simulink model "MPC"  (R2020a)
settings: Solver=ode4  StartTime=0.0  StopTime=200  FixedStep=1  RelTol=1e-3
InitFcn:
  | SetupParameters
StopFcn:
  | PlotResults
values from neighbouring files (symbols this model uses):
  A = reshape(Aflat,n,n)    [mpc_s_L2.m]    (also in prediction.m = delayMod.A)
  B1 = reshape(B1flat,n,[])    [mpc_s_L2.m]    (also in prediction.m = delayMod.B1)
  CforStateOutput = eye(4)    [SetupParameters.m]    (also in TestMPC.m)
  DforStateOutput = zeros(n, p)    [SetupParameters.m]    (also in TestMPC.m)
  G = [G11 G12; G21 G22]    [SetupParameters.m]    (also in TestMPC.m)
  plantD = ss(Gd)    [SetupParameters.m]    (also in TestMPC.m; mpc_s_L2.m)
  tau = block.Dwork(11).Data    [mpc_s_L2.m]    (also in prediction.m = delayMod.tau)
  Ts = 1    [SetupParameters.m]    (also in TestMPC.m; mpc_s_L2.m = block.DialogPrm(8).Data)
undefined symbols (not defined in the file or in its folder): H
settings Model: Creator=Charl  LastModifiedBy=Charl

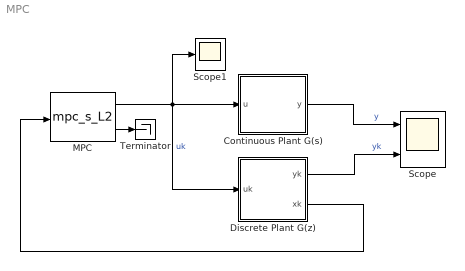
== system MPC ==
  Continuous Plant G(s) : Subsystem
  Discrete Plant G(z) : Subsystem
  MPC : M-S-Function  FunctionName=mpc_s_L2  Parameters=Gd, Ysp, Np, Nb, Nc, Q, R, Ts
  Scope : Scope  NumInputPorts=2
  Scope1 : Scope
  Terminator : Terminator
  wires:
  Continuous Plant G(s)/1(y) -> Scope/1  "y"
  MPC/1 -> Scope1/1, Discrete Plant G(z)/1(uk), Continuous Plant G(s)/1(u)  "uk"
  MPC/2 -> Terminator/1
  Discrete Plant G(z)/2(xk) -> MPC/1
  Discrete Plant G(z)/1(yk) -> Scope/2  "yk"

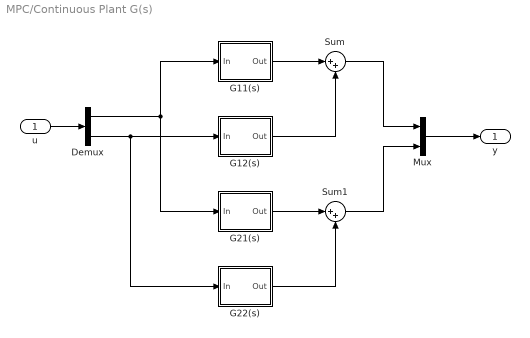
== system MPC/Continuous Plant G(s) ==
  u : Inport
  Demux : Demux  Outputs=2
  G11(s) : Subsystem
  G12(s) : Subsystem
  G21(s) : Subsystem
  G22(s) : Subsystem
  Mux : Mux  Inputs=2
  Sum : Sum  Inputs=|++
  Sum1 : Sum  Inputs=|++
  y : Outport
  wires:
  G11(s)/1(Out) -> Sum/1
  G22(s)/1(Out) -> Sum1/2
  G21(s)/1(Out) -> Sum1/1
  G12(s)/1(Out) -> Sum/2
  Demux/1 -> G11(s)/1(In), G21(s)/1(In)
  Demux/2 -> G22(s)/1(In), G12(s)/1(In)
  u/1 -> Demux/1
  Sum/1 -> Mux/1
  Sum1/1 -> Mux/2
  Mux/1 -> y/1

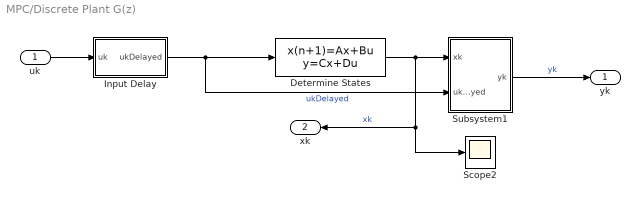
== system MPC/Discrete Plant G(z) ==
  uk : Inport
  Determine States : DiscreteStateSpace  A=A  B=B1  C=CforStateOutput  D=DforStateOutput  SampleTime=Ts
  Input Delay : Subsystem
  Scope2 : Scope
  Subsystem1 : Subsystem
  yk : Outport
  xk : Outport  Port=2
  wires:
  Input Delay/1(ukDelayed) -> Determine States/1, Subsystem1/2(ukDelayed)  "ukDelayed"
  uk/1 -> Input Delay/1(uk)
  Determine States/1 -> xk/1, Scope2/1, Subsystem1/1(xk)  "xk"
  Subsystem1/1(yk) -> yk/1  "yk"

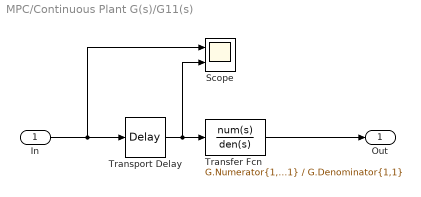
== system MPC/Continuous Plant G(s)/G11(s) ==
  In : Inport
  Scope : Scope  NumInputPorts=2
  Transfer Fcn : TransferFcn  Numerator=G.Numerator{1,1}  Denominator=G.Denominator{1,1}
  Transport Delay : TransportDelay  DelayTime=G.IODelay(1,1)
  Out : Outport
  wires:
  Transfer Fcn/1 -> Out/1
  In/1 -> Scope/1, Transport Delay/1
  Transport Delay/1 -> Scope/2, Transfer Fcn/1

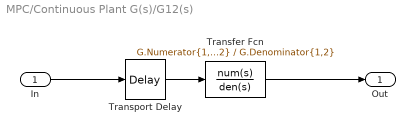
== system MPC/Continuous Plant G(s)/G12(s) ==
  In : Inport
  Transfer Fcn : TransferFcn  Numerator=G.Numerator{1,2}  Denominator=G.Denominator{1,2}
  Transport Delay : TransportDelay  DelayTime=G.IODelay(1,2)
  Out : Outport
  wires:
  Transport Delay/1 -> Transfer Fcn/1
  Transfer Fcn/1 -> Out/1
  In/1 -> Transport Delay/1

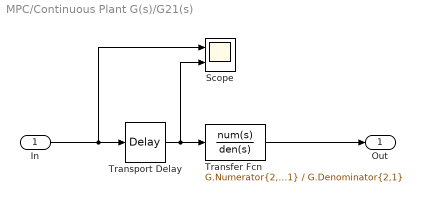
== system MPC/Continuous Plant G(s)/G21(s) ==
  In : Inport
  Scope : Scope  NumInputPorts=2
  Transfer Fcn : TransferFcn  Numerator=G.Numerator{2,1}  Denominator=G.Denominator{2,1}
  Transport Delay : TransportDelay  DelayTime=G.IODelay(2,1)
  Out : Outport
  wires:
  Transport Delay/1 -> Scope/2, Transfer Fcn/1
  Transfer Fcn/1 -> Out/1
  In/1 -> Scope/1, Transport Delay/1

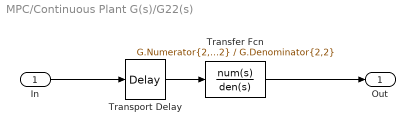
== system MPC/Continuous Plant G(s)/G22(s) ==
  In : Inport
  Transfer Fcn : TransferFcn  Numerator=G.Numerator{2,2}  Denominator=G.Denominator{2,2}
  Transport Delay : TransportDelay  DelayTime=G.IODelay(2,2)
  Out : Outport
  wires:
  Transport Delay/1 -> Transfer Fcn/1
  Transfer Fcn/1 -> Out/1
  In/1 -> Transport Delay/1

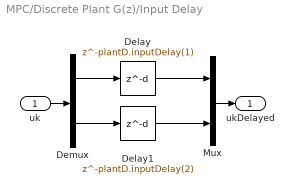
== system MPC/Discrete Plant G(z)/Input Delay ==
  uk : Inport
  Delay : Delay  DelayLength=plantD.inputDelay(1)  SampleTime=Ts
  Delay1 : Delay  DelayLength=plantD.inputDelay(2)
  Demux : Demux  Outputs=2
  Mux : Mux  Inputs=2
  ukDelayed : Outport
  wires:
  Demux/1 -> Delay/1
  Delay/1 -> Mux/1
  Mux/1 -> ukDelayed/1
  Demux/2 -> Delay1/1
  Delay1/1 -> Mux/2
  uk/1 -> Demux/1

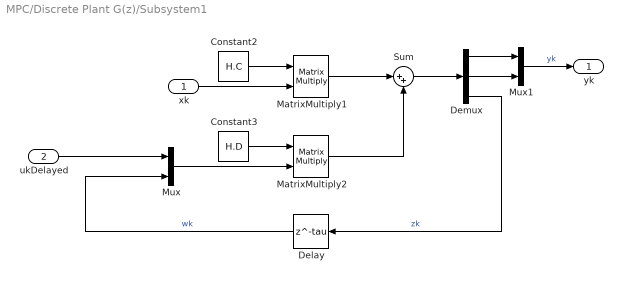
== system MPC/Discrete Plant G(z)/Subsystem1 ==
  xk : Inport
  ukDelayed : Inport  Port=2
  Constant2 : Constant  Value=H.C  VectorParams1D=off
  Constant3 : Constant  Value=H.D  VectorParams1D=off
  Delay : Delay  DelayLength=tau
  Demux : Demux  Outputs=3
  MatrixMultiply1 : Product  Multiplication=Matrix(*)
  MatrixMultiply2 : Product  Multiplication=Matrix(*)
  Mux : Mux  Inputs=2
  Mux1 : Mux  Inputs=2
  Sum : Sum  Inputs=|++
  yk : Outport
  wires:
  MatrixMultiply1/1 -> Sum/1
  Sum/1 -> Demux/1
  Demux/2 -> Mux1/2
  Demux/3 -> Delay/1  "zk"
  Constant3/1 -> MatrixMultiply2/1
  Delay/1 -> Mux/2  "wk"
  MatrixMultiply2/1 -> Sum/2
  Constant2/1 -> MatrixMultiply1/1
  Demux/1 -> Mux1/1
  Mux/1 -> MatrixMultiply2/2
  xk/1 -> MatrixMultiply1/2
  ukDelayed/1 -> Mux/1
  Mux1/1 -> yk/1  "yk"
